simulink model "shaping_filter"  (R2015a)
settings: Solver=ode45  StartTime=0.0  StopTime=10.0  RelTol=1e-3
libraries: simulink_extras x2
settings Model: Creator=ayush  LastModifiedBy=ayush

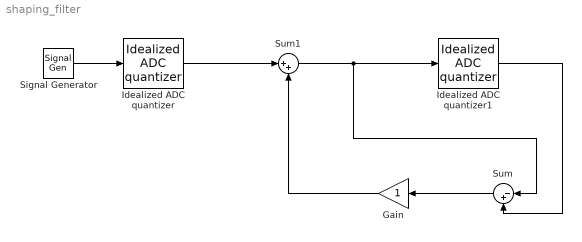
== system shaping_filter ==
  Gain : Gain
  Idealized ADC quantizer : simulink_extras/Additional Discrete/Idealized ADC quantizer  NumberOfConverterBits=16  Vmin=0  Vmax=5  OutputDataType=double  OutputNegativeValues=on
  Idealized ADC quantizer1 : simulink_extras/Additional Discrete/Idealized ADC quantizer  NumberOfConverterBits=12  Vmin=0  Vmax=5  OutputDataType=double  OutputNegativeValues=on
  Signal Generator : SignalGenerator  WaveForm=sawtooth  Frequency=100
  Sum : Sum  Inputs=|-+
  Sum1 : Sum  Inputs=|++
  wires:
  Sum/1 -> Gain/1
  Idealized ADC quantizer/1 -> Sum1/1
  Gain/1 -> Sum1/2
  Sum1/1 -> Sum/1, Idealized ADC quantizer1/1
  Idealized ADC quantizer1/1 -> Sum/2
  Signal Generator/1 -> Idealized ADC quantizer/1
